simulink model "Model_ukladu_kociol_turbina"  (Simulink 7.9)
settings: Solver=ode45  StartTime=0.0  StopTime=3500  RelTol=1e-3
settings Model: Creator=Ja  LastModifiedBy=Ja

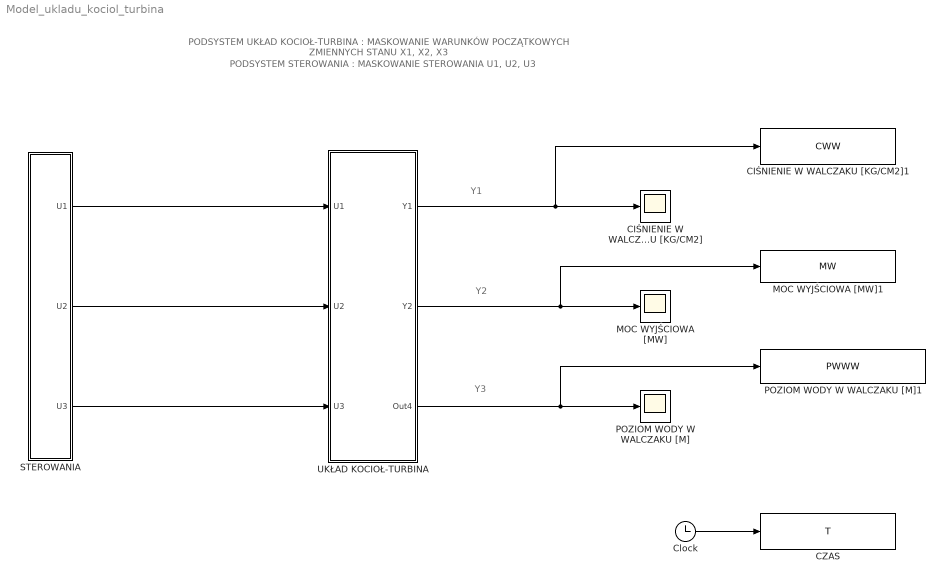
== system Model_ukladu_kociol_turbina ==
  note: Y1
  note: Y2
  note: Y3
  note: PODSYSTEM UKŁAD KOCIOŁ-TURBINA : MASKOWANIE WARUNKÓW POCZĄTKOWYCH ZMIENNYCH STANU X1, X2, X3
  note: PODSYSTEM STEROWANIA : MASKOWANIE STEROWANIA U1, U2, U3
  CIŚNIENIE W WALCZAKU [KG/CM2] : Scope
      settings: RequirementInfo="{}  %GIDa_61236fcf_196b_432a_8315_ec735b276141"
  CIŚNIENIE W WALCZAKU [KG/CM2]1 : ToWorkspace  VariableName=CWW  SampleTime=-1  SaveFormat=Timeseries
  CZAS : ToWorkspace  VariableName=T  SampleTime=-1  SaveFormat=Timeseries
  Clock : Clock
  MOC WYJŚCIOWA [MW] : Scope
      settings: SaveName=ScopeData2
  MOC WYJŚCIOWA [MW]1 : ToWorkspace  VariableName=MW  SampleTime=-1  SaveFormat=Timeseries
  POZIOM WODY W WALCZAKU [M] : Scope
      settings: SaveName=ScopeData4
  POZIOM WODY W WALCZAKU [M]1 : ToWorkspace  VariableName=PWWW  SampleTime=-1  SaveFormat=Timeseries
  STEROWANIA : Subsystem  mask{u1o=0.271, u1=0.371, u2o=0.621, u2=0.621, u3o=0.34, u3=0.34, ts=500}
      mask prompts: u1o "OTWARCIE ZAWORU PALIWA [POCZ.]"; u1 "OTWARCIE ZAWORU PALIWA [KONC.]"; u2o "ZNORMALIZOWANY PRZEPŁYW PARY [POCZ.]"; u2 "ZNORMALIZOWANY PRZEPŁYW PARY [KONC.]"; u3o "ZNORMALIZOWANY PRZEPŁYW WODY ZASILAJĄCEJ [POCZ.]"; u3 "ZNORMALIZOWANY PRZEPŁYW WODY ZASILAJĄCEJ [KONC.]"; ts "CZAS SKOKU"
  UKŁAD KOCIOŁ-TURBINA : Subsystem  mask{S1=97.20, S2=50.52, S3=385.2}
      mask prompts: S1 "WARUNEK POCZĄTKOWY X1"; S2 "WARUNEK POCZĄTKOWY X2"; S3 "WARUNEK POCZĄTKOWY X3"
  wires:
  UKŁAD KOCIOŁ-TURBINA/2(Y2) -> MOC WYJŚCIOWA [MW]/1, MOC WYJŚCIOWA [MW]1/1
  UKŁAD KOCIOŁ-TURBINA/3(Out4) -> POZIOM WODY W WALCZAKU [M]/1, POZIOM WODY W WALCZAKU [M]1/1
  UKŁAD KOCIOŁ-TURBINA/1(Y1) -> CIŚNIENIE W WALCZAKU [KG/CM2]/1, CIŚNIENIE W WALCZAKU [KG/CM2]1/1
  STEROWANIA/1(U1) -> UKŁAD KOCIOŁ-TURBINA/1(U1)
  STEROWANIA/2(U2) -> UKŁAD KOCIOŁ-TURBINA/2(U2)
  STEROWANIA/3(U3) -> UKŁAD KOCIOŁ-TURBINA/3(U3)
  Clock/1 -> CZAS/1

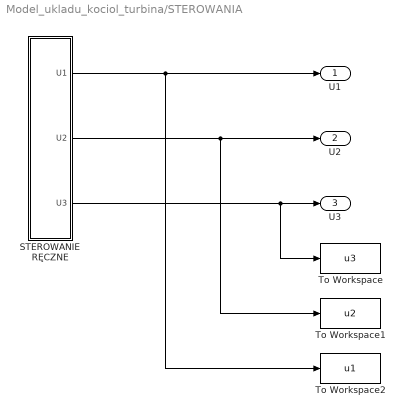
== system Model_ukladu_kociol_turbina/STEROWANIA ==
  STEROWANIE RĘCZNE : Subsystem
  To Workspace : ToWorkspace  VariableName=u3  SampleTime=-1  SaveFormat=Timeseries
  To Workspace1 : ToWorkspace  VariableName=u2  SampleTime=-1  SaveFormat=Timeseries
  To Workspace2 : ToWorkspace  VariableName=u1  SampleTime=-1  SaveFormat=Timeseries
  U1 : Outport
  U2 : Outport  Port=2
  U3 : Outport  Port=3
  wires:
  STEROWANIE RĘCZNE/3(U3) -> U3/1, To Workspace/1
  STEROWANIE RĘCZNE/2(U2) -> U2/1, To Workspace1/1
  STEROWANIE RĘCZNE/1(U1) -> U1/1, To Workspace2/1

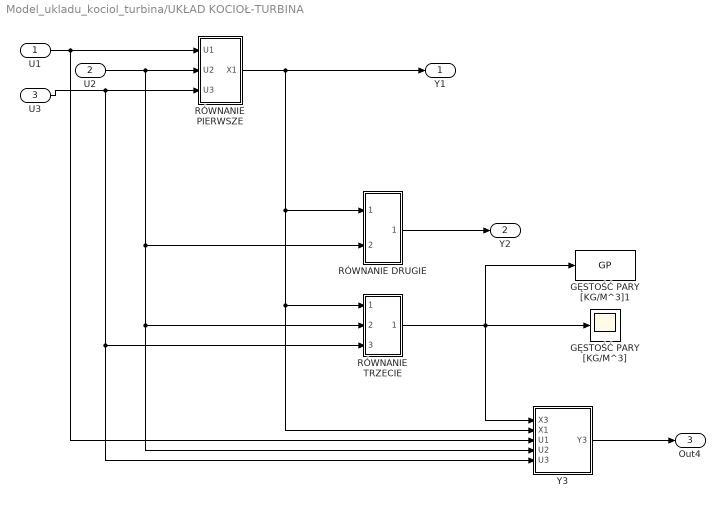
== system Model_ukladu_kociol_turbina/UKŁAD KOCIOŁ-TURBINA ==
  U1 : Inport
  U2 : Inport  Port=2
  U3 : Inport  Port=3
  GĘSTOŚĆ PARY [KG/M^3] : Scope
  GĘSTOŚĆ PARY [KG/M^3]1 : ToWorkspace  VariableName=GP  SampleTime=-1  SaveFormat=Timeseries
  RÓWNANIE DRUGIE : Subsystem
  RÓWNANIE PIERWSZE : Subsystem
  RÓWNANIE TRZECIE : Subsystem
  Y3 : Subsystem  mask{warunek=0}
      mask prompts: warunek "TYLKO >= 0  DLA Y3 (0 WYL)"
  Y1 : Outport
  Y2 : Outport  Port=2
  Out4 : Outport  Port=3
  wires:
  U2/1 -> Y3/4(U2), RÓWNANIE TRZECIE/2(U2), RÓWNANIE DRUGIE/2(U2), RÓWNANIE PIERWSZE/2(U2)
  U1/1 -> Y3/3(U1), RÓWNANIE PIERWSZE/1(U1)
  U3/1 -> Y3/5(U3), RÓWNANIE TRZECIE/3(U3), RÓWNANIE PIERWSZE/3(U3)
  RÓWNANIE PIERWSZE/1(X1) -> RÓWNANIE DRUGIE/1(X1), RÓWNANIE TRZECIE/1(X1), Y3/2(X1), Y1/1
  RÓWNANIE TRZECIE/1(X3) -> Y3/1(X3), GĘSTOŚĆ PARY [KG/M^3]/1, GĘSTOŚĆ PARY [KG/M^3]1/1
  RÓWNANIE DRUGIE/1(X2) -> Y2/1
  Y3/1(Y3) -> Out4/1

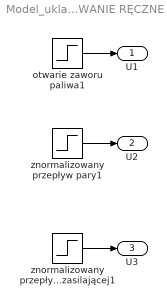
== system Model_ukladu_kociol_turbina/STEROWANIA/STEROWANIE RĘCZNE ==
  otwarie zaworu paliwa1 : Step  Time=ts  Before=u1o  After=u1  SampleTime=0
  znormalizowany przepływ pary1 : Step  Time=ts  Before=u2o  After=u2  SampleTime=0
  znormalizowany przepływ wody zasilającej1 : Step  Time=ts  Before=u3o  After=u3  SampleTime=0
  U1 : Outport
  U2 : Outport  Port=2
  U3 : Outport  Port=3
  wires:
  znormalizowany przepływ wody zasilającej1/1 -> U3/1
  znormalizowany przepływ pary1/1 -> U2/1
  otwarie zaworu paliwa1/1 -> U1/1

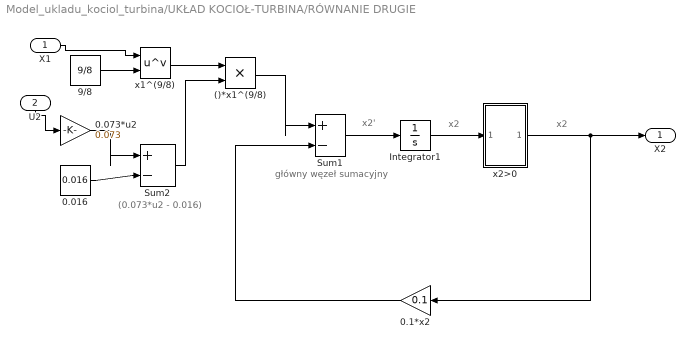
== system Model_ukladu_kociol_turbina/UKŁAD KOCIOŁ-TURBINA/RÓWNANIE DRUGIE ==
  note: x2'
  note: x2
  note: (0.073*u2 - 0.016)
  note: główny węzeł sumacyjny
  note: x2
  X1 : Inport
  U2 : Inport  Port=2
  ()*x1^(9/8) : Product  RndMeth=Zero
  0.016 : Constant  Value=0.016
  0.073*u2 : Gain  Gain=0.073
  0.1*x2 : Gain  Gain=0.1
  9/8 : Constant  Value=9/8
  Integrator1 : Integrator  InitialCondition=S2
  Sum1 : Sum  Inputs=|+-
  Sum2 : Sum  Inputs=|+-
  x1^(9/8) : Math  Operator=pow  SaturateOnIntegerOverflow=on
  x2>0 : Subsystem
  X2 : Outport
  wires:
  Sum1/1 -> Integrator1/1
  0.1*x2/1 -> Sum1/2
  9/8/1 -> x1^(9/8)/2
  x1^(9/8)/1 -> ()*x1^(9/8)/1
  ()*x1^(9/8)/1 -> Sum1/1
  Sum2/1 -> ()*x1^(9/8)/2
  0.016/1 -> Sum2/2
  0.073*u2/1 -> Sum2/1
  X1/1 -> x1^(9/8)/1
  U2/1 -> 0.073*u2/1
  x2>0/1(Out1) -> X2/1, 0.1*x2/1
  Integrator1/1 -> x2>0/1(In1)

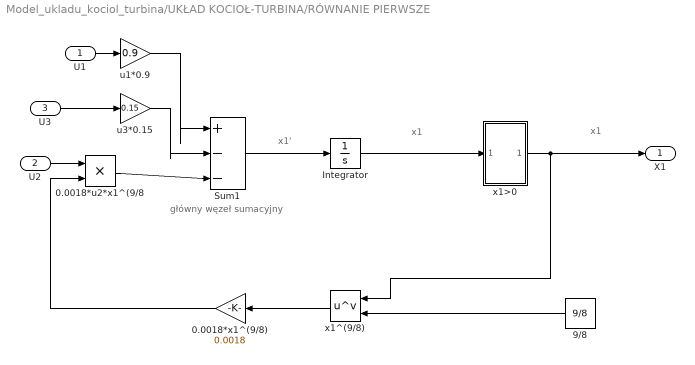
== system Model_ukladu_kociol_turbina/UKŁAD KOCIOŁ-TURBINA/RÓWNANIE PIERWSZE ==
  note: x1'
  note: x1
  note: główny węzeł sumacyjny
  note: x1
  U1 : Inport
  U2 : Inport  Port=2
  U3 : Inport  Port=3
  0.0018*u2*x1^(9/8 : Product  RndMeth=Zero
  0.0018*x1^(9/8) : Gain  Gain=0.0018
  9/8 : Constant  Value=9/8
  Integrator : Integrator  InitialCondition=S1
  Sum1 : Sum  Inputs=|+--
  u1*0.9 : Gain  Gain=0.9
  u3*0.15 : Gain  Gain=0.15
  x1>0 : Subsystem
  x1^(9/8) : Math  Operator=pow  SaturateOnIntegerOverflow=on
  X1 : Outport
  wires:
  Sum1/1 -> Integrator/1
  9/8/1 -> x1^(9/8)/2
  x1^(9/8)/1 -> 0.0018*x1^(9/8)/1
  0.0018*x1^(9/8)/1 -> 0.0018*u2*x1^(9/8/2
  0.0018*u2*x1^(9/8/1 -> Sum1/3
  u1*0.9/1 -> Sum1/1
  u3*0.15/1 -> Sum1/2
  U1/1 -> u1*0.9/1
  U3/1 -> u3*0.15/1
  U2/1 -> 0.0018*u2*x1^(9/8/1
  x1>0/1(Out1) -> X1/1, x1^(9/8)/1
  Integrator/1 -> x1>0/1(In1)

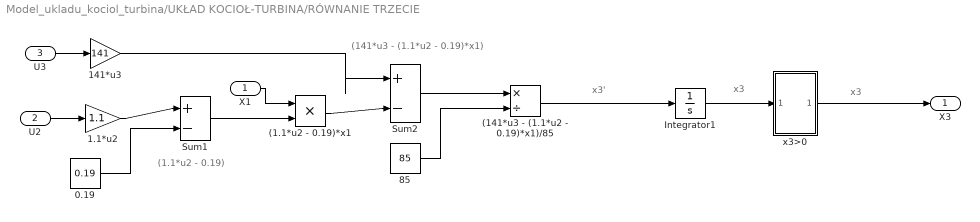
== system Model_ukladu_kociol_turbina/UKŁAD KOCIOŁ-TURBINA/RÓWNANIE TRZECIE ==
  note: (141*u3 - (1.1*u2 - 0.19)*x1)
  note: (1.1*u2 - 0.19)
  note: x3
  note: x3'
  note: x3
  X1 : Inport
  U2 : Inport  Port=2
  U3 : Inport  Port=3
  (1.1*u2 - 0.19)*x1 : Product  RndMeth=Zero
  (141*u3 - (1.1*u2 - 0.19)*x1)/85 : Product  Inputs=*/
  0.19 : Constant  Value=0.19
  1.1*u2 : Gain  Gain=1.1
  141*u3 : Gain  Gain=141
  85 : Constant  Value=85
  Integrator1 : Integrator  InitialCondition=S3
  Sum1 : Sum  Inputs=|+-
  Sum2 : Sum  Inputs=|+-
  x3>0 : Subsystem
  X3 : Outport
  wires:
  (141*u3 - (1.1*u2 - 0.19)*x1)/85/1 -> Integrator1/1
  Sum2/1 -> (141*u3 - (1.1*u2 - 0.19)*x1)/85/1
  85/1 -> (141*u3 - (1.1*u2 - 0.19)*x1)/85/2
  141*u3/1 -> Sum2/1
  (1.1*u2 - 0.19)*x1/1 -> Sum2/2
  Sum1/1 -> (1.1*u2 - 0.19)*x1/2
  0.19/1 -> Sum1/2
  1.1*u2/1 -> Sum1/1
  U3/1 -> 141*u3/1
  X1/1 -> (1.1*u2 - 0.19)*x1/1
  U2/1 -> 1.1*u2/1
  x3>0/1(Out1) -> X3/1
  Integrator1/1 -> x3>0/1(In1)

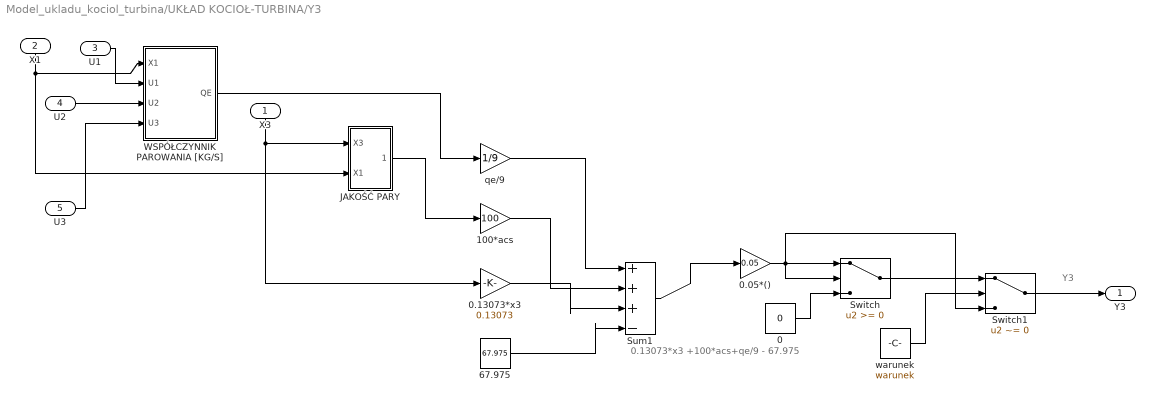
== system Model_ukladu_kociol_turbina/UKŁAD KOCIOŁ-TURBINA/Y3 ==
  note: 0.13073*x3 +100*acs+qe/9 - 67.975
  note: Y3
  X3 : Inport
  X1 : Inport  Port=2
  U1 : Inport  Port=3
  U2 : Inport  Port=4
  U3 : Inport  Port=5
  0 : Constant  Value=0
  0.05*() : Gain  Gain=0.05
  0.13073*x3 : Gain  Gain=0.13073
  100*acs : Gain  Gain=100
  67.975 : Constant  Value=67.975
  JAKOŚĆ PARY : Subsystem
  Sum1 : Sum  Inputs=|+++-
  Switch : Switch
  Switch1 : Switch  Criteria=u2 ~= 0
  WSPÓŁCZYNNIK PAROWANIA [KG/S] : Subsystem
  qe/9 : Gain  Gain=1/9
  warunek : Constant  Value=warunek
  Y3 : Outport
  wires:
  JAKOŚĆ PARY/1(ACS) -> 100*acs/1
  WSPÓŁCZYNNIK PAROWANIA [KG/S]/1(QE) -> qe/9/1
  67.975/1 -> Sum1/4
  0.13073*x3/1 -> Sum1/3
  100*acs/1 -> Sum1/2
  qe/9/1 -> Sum1/1
  Sum1/1 -> 0.05*()/1
  X1/1 -> WSPÓŁCZYNNIK PAROWANIA [KG/S]/1(X1), JAKOŚĆ PARY/2(X1)
  U1/1 -> WSPÓŁCZYNNIK PAROWANIA [KG/S]/2(U1)
  U2/1 -> WSPÓŁCZYNNIK PAROWANIA [KG/S]/3(U2)
  U3/1 -> WSPÓŁCZYNNIK PAROWANIA [KG/S]/4(U3)
  X3/1 -> 0.13073*x3/1, JAKOŚĆ PARY/1(X3)
  0.05*()/1 -> Switch/2, Switch/1, Switch1/3
  0/1 -> Switch/3
  Switch1/1 -> Y3/1
  warunek/1 -> Switch1/2
  Switch/1 -> Switch1/1

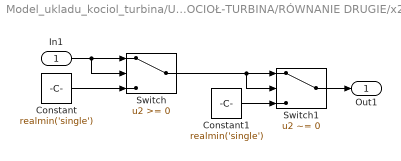
== system Model_ukladu_kociol_turbina/UKŁAD KOCIOŁ-TURBINA/RÓWNANIE DRUGIE/x2>0 ==
  In1 : Inport
  Constant : Constant  Value=realmin('single')
  Constant1 : Constant  Value=realmin('single')
  Switch : Switch
  Switch1 : Switch  Criteria=u2 ~= 0
  Out1 : Outport
  wires:
  Constant/1 -> Switch/3
  Constant1/1 -> Switch1/3
  Switch/1 -> Switch1/1, Switch1/2
  In1/1 -> Switch/2, Switch/1
  Switch1/1 -> Out1/1

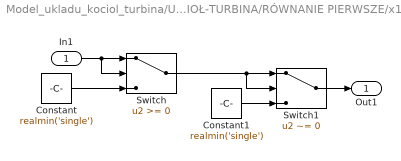
== system Model_ukladu_kociol_turbina/UKŁAD KOCIOŁ-TURBINA/RÓWNANIE PIERWSZE/x1>0 ==
  In1 : Inport
  Constant : Constant  Value=realmin('single')
  Constant1 : Constant  Value=realmin('single')
  Switch : Switch
  Switch1 : Switch  Criteria=u2 ~= 0
  Out1 : Outport
  wires:
  Constant/1 -> Switch/3
  Constant1/1 -> Switch1/3
  Switch/1 -> Switch1/1, Switch1/2
  In1/1 -> Switch/2, Switch/1
  Switch1/1 -> Out1/1

== system Model_ukladu_kociol_turbina/UKŁAD KOCIOŁ-TURBINA/RÓWNANIE TRZECIE/x3>0 ==
  In1 : Inport
  Constant : Constant  Value=realmin('single')
  Constant1 : Constant  Value=realmin('single')
  Switch : Switch
  Switch1 : Switch  Criteria=u2 ~= 0
  Out1 : Outport
  wires:
  Constant/1 -> Switch/3
  Constant1/1 -> Switch1/3
  Switch/1 -> Switch1/1, Switch1/2
  In1/1 -> Switch/2, Switch/1
  Switch1/1 -> Out1/1

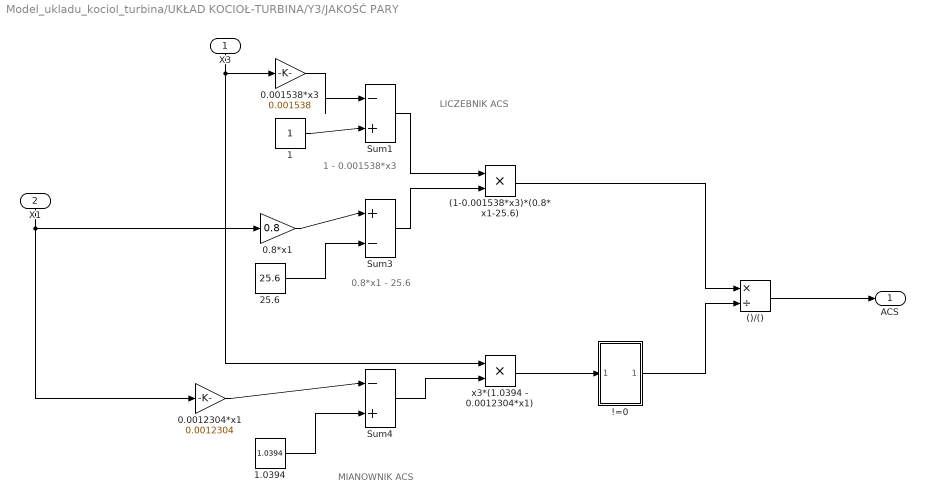
== system Model_ukladu_kociol_turbina/UKŁAD KOCIOŁ-TURBINA/Y3/JAKOŚĆ PARY ==
  note: 1 - 0.001538*x3
  note: 0.8*x1 - 25.6
  note: LICZEBNIK ACS
  note: MIANOWNIK ACS
  X3 : Inport
  X1 : Inport  Port=2
  !=0 : Subsystem
  ()/() : Product  Inputs=*/
  (1-0.001538*x3)*(0.8*x1-25.6) : Product  RndMeth=Zero
  0.0012304*x1 : Gain  Gain=0.0012304
  0.001538*x3 : Gain  Gain=0.001538
  0.8*x1 : Gain  Gain=0.8
  1 : Constant
  1.0394 : Constant  Value=1.0394
  25.6 : Constant  Value=25.6
  Sum1 : Sum  Inputs=|-+
  Sum3 : Sum  Inputs=|+-
  Sum4 : Sum  Inputs=|-+
  x3*(1.0394 - 0.0012304*x1) : Product  RndMeth=Zero
  ACS : Outport
  wires:
  1/1 -> Sum1/2
  0.001538*x3/1 -> Sum1/1
  0.8*x1/1 -> Sum3/1
  25.6/1 -> Sum3/2
  Sum3/1 -> (1-0.001538*x3)*(0.8*x1-25.6)/2
  Sum1/1 -> (1-0.001538*x3)*(0.8*x1-25.6)/1
  0.0012304*x1/1 -> Sum4/1
  1.0394/1 -> Sum4/2
  Sum4/1 -> x3*(1.0394 - 0.0012304*x1)/2
  ()/()/1 -> ACS/1
  X3/1 -> 0.001538*x3/1, x3*(1.0394 - 0.0012304*x1)/1
  X1/1 -> 0.8*x1/1, 0.0012304*x1/1
  x3*(1.0394 - 0.0012304*x1)/1 -> !=0/1(In1)
  !=0/1(Out1) -> ()/()/2
  (1-0.001538*x3)*(0.8*x1-25.6)/1 -> ()/()/1

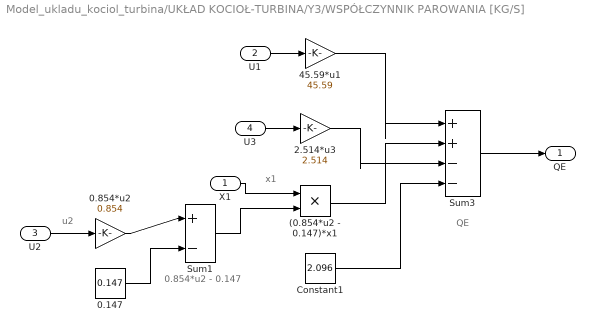
== system Model_ukladu_kociol_turbina/UKŁAD KOCIOŁ-TURBINA/Y3/WSPÓŁCZYNNIK PAROWANIA [KG/S] ==
  note: 0.854*u2 - 0.147
  note: x1
  note: u2
  note: QE
  X1 : Inport
  U1 : Inport  Port=2
  U2 : Inport  Port=3
  U3 : Inport  Port=4
  (0.854*u2 - 0.147)*x1 : Product  RndMeth=Zero
  0.147 : Constant  Value=0.147
  0.854*u2 : Gain  Gain=0.854
  2.514*u3 : Gain  Gain=2.514
  45.59*u1 : Gain  Gain=45.59
  Constant1 : Constant  Value=2.096
  Sum1 : Sum  Inputs=|+-
  Sum3 : Sum  Inputs=|++--
  QE : Outport
  wires:
  0.854*u2/1 -> Sum1/1
  0.147/1 -> Sum1/2
  Sum1/1 -> (0.854*u2 - 0.147)*x1/2
  45.59*u1/1 -> Sum3/1
  (0.854*u2 - 0.147)*x1/1 -> Sum3/2
  2.514*u3/1 -> Sum3/3
  Constant1/1 -> Sum3/4
  Sum3/1 -> QE/1
  U1/1 -> 45.59*u1/1
  U3/1 -> 2.514*u3/1
  X1/1 -> (0.854*u2 - 0.147)*x1/1
  U2/1 -> 0.854*u2/1

== system Model_ukladu_kociol_turbina/UKŁAD KOCIOŁ-TURBINA/Y3/JAKOŚĆ PARY/!=0 ==
  In1 : Inport
  Constant1 : Constant  Value=realmin('single')
  Switch1 : Switch  Criteria=u2 ~= 0
  Out1 : Outport
  wires:
  Constant1/1 -> Switch1/3
  Switch1/1 -> Out1/1
  In1/1 -> Switch1/1, Switch1/2
